simulink model "test_writer"  (R2021a)
settings: Solver=FixedStepAuto  StartTime=0.0  StopTime=10.0  RelTol=1e-3
libraries: ddsblock x1
settings Model: DataDictionary=test_writer.sldd  Creator=leon  LastModifiedBy=leon
settings OptimizationCC: DefaultParameterBehavior=Inlined  EnhancedBackFolding=on  PassReuseOutputArgsAs=Individual arguments  ZeroExternalMemoryAtStartup=off  ZeroInternalMemoryAtStartup=off  OptimizeBlockOrder=speed  DifferentSizesBufferReuse=on  OptimizationCustomize=off  EfficientTunableParamExpr=on
settings DebuggingCC: ParameterTunabilityLossMsg=error
settings SFSimCC: SimGenImportedTypeDefs=on  MATLABDynamicMemAlloc=off
settings RTWCC: SystemTargetFile=ert.tlc  TemplateMakefile=ert_default_tmf  Toolchain=eProsima 1.8 Project  TargetLang=C++
settings CodeAppCC: ForceParamTrailComments=on  IgnoreCustomStorageClasses=off  OperatorAnnotations=on  SimulinkDataObjDesc=on  SFDataObjDesc=on  InsertBlockDesc=on
settings ERTTargetCC: TargetLangStandard=C++11 (ISO)  CodeInterfacePackaging=C++ class  InlinedParameterPlacement=NonHierarchical  RootIOFormat=Structure reference  ERTCustomFileTemplate=example_file_process.tlc  ArrayContainerType=std::array

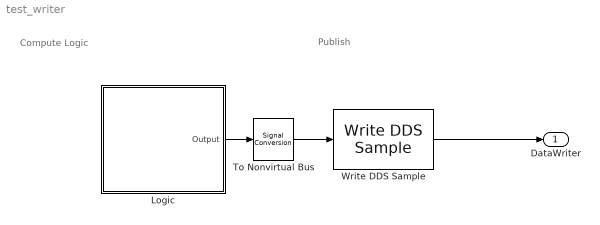
== system test_writer ==
  note: Publish
  note: Compute Logic
  Logic : Subsystem
  To Nonvirtual Bus : SignalConversion  ConversionOutput=Nonvirtual bus  OverrideOpt=off
  Write DDS Sample : ddsblock/Write DDS Sample
      settings: SourceProductBaseCode=DD
  DataWriter : Outport  InputPortMessageModes=m  OutDataTypeStr=Bus: HLCHello  BusOutputAsStruct=on
  wires:
  Write DDS Sample/1 -> DataWriter/1
  Logic/1(Output) -> To Nonvirtual Bus/1
  To Nonvirtual Bus/1 -> Write DDS Sample/1

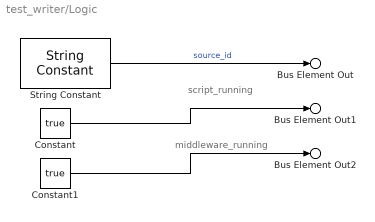
== system test_writer/Logic ==
  note: middleware_running
  note: script_running
  Constant : Constant  Value=true
  Constant1 : Constant  Value=true
  String Constant : StringConstant  String="\"Test\""
  Bus Element Out : Outport  PortName=Output  Element=source_id
  Bus Element Out1 : Outport  PortName=Output  Element=script_running
  Bus Element Out2 : Outport  PortName=Output  Element=middleware_running
  wires:
  String Constant/1 -> Bus Element Out/1  "source_id"
  Constant/1 -> Bus Element Out1/1
  Constant1/1 -> Bus Element Out2/1
